simulink model "adaptive_control_sim"  (R2020a)
settings: Solver=FixedStepAuto  StartTime=0.0  StopTime=T  FixedStep=dtmax  MaxStep=dtmax  RelTol=1e-3
values from neighbouring files (symbols this model uses):
  b = b*b_error_scale    (= 131.4)    [Hinf_run.m]    (also in adaptive_control_run.m; passivity_fmod_run.m; passivity_velmod_run.m)
  bhat = 100    [adaptive_control_run.m]
  fe_dz = 15    [adaptive_control_run.m]
  input_type = 3    [Hinf_run.m]    (also in adaptive_control_run.m; passivity_fmod_run.m; passivity_velmod_run.m)
  k = k*k_error_scale    (= 11691)    [Hinf_run.m]    (also in adaptive_control_run.m; passivity_fmod_run.m; passivity_velmod_run.m)
  Kb = 40    [adaptive_control_run.m]
  khat = 11000    [adaptive_control_run.m]
  KK = 40    [adaptive_control_run.m]
  m = 500    [Hinf_run.m]    (also in adaptive_control_run.m; passivity_fmod_run.m; passivity_velmod_run.m)
  rampslope = 0.1    [Hinf_run.m]    (also in adaptive_control_run.m; passivity_fmod_run.m; passivity_velmod_run.m)
  sineamp = 0.1    [Hinf_run.m]    (also in adaptive_control_run.m; passivity_fmod_run.m; passivity_velmod_run.m)
  sinefreq = pi/2    (= 1.57079632679)    [Hinf_run.m]    (also in adaptive_control_run.m; passivity_fmod_run.m; passivity_velmod_run.m)
  stepval = 0.1    [Hinf_run.m]    (also in adaptive_control_run.m; passivity_fmod_run.m; passivity_velmod_run.m)
  taum = taum*taum_error_scale    (= 0.108)    [Hinf_run.m]    (also in adaptive_control_run.m; passivity_fmod_run.m; passivity_velmod_run.m)
  taumreal = 1*taum    (= 0.108)    [adaptive_control_run.m]
settings Model: Creator=davidcarabis  LastModifiedBy=davidcarabis
settings DataIOCC: ReturnWorkspaceOutputs=off

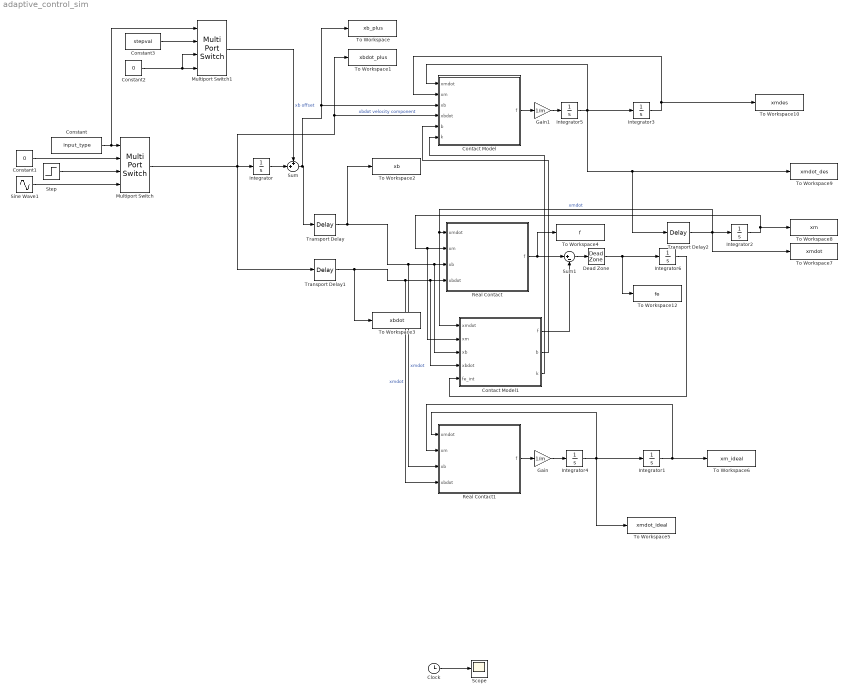
== system adaptive_control_sim ==
  Clock : Clock
  Constant : Constant  Value=input_type
  Constant1 : Constant  Value=0
  Constant2 : Constant  Value=0
  Constant3 : Constant  Value=stepval
  Contact Model : Subsystem
  Contact Model1 : Subsystem
  Dead Zone : DeadZone  LowerValue=-fe_dz  UpperValue=fe_dz  SaturateOnIntegerOverflow=on
  Gain : Gain  Gain=1/m
  Gain1 : Gain  Gain=1/m
  Integrator{,1..6} (7 alike) : Integrator
  Multiport Switch : MultiPortSwitch
  Multiport Switch1 : MultiPortSwitch
  Real Contact : Subsystem
  Real Contact1 : Subsystem
  Scope : Scope
  Sine Wave1 : Sin  Amplitude=sineamp*sinefreq  Frequency=sinefreq  Phase=pi/2  SampleTime=0
  Step : Step  Time=0  After=rampslope  SampleTime=0
  Sum : Sum  Inputs=++|
  Sum1 : Sum  Inputs=|+-
  To Workspace : ToWorkspace  VariableName=xb_plus
  To Workspace1 : ToWorkspace  VariableName=xbdot_plus
  To Workspace10 : ToWorkspace  VariableName=xmdes
  To Workspace12 : ToWorkspace  VariableName=fe
  To Workspace2 : ToWorkspace  VariableName=xb
  To Workspace3 : ToWorkspace  VariableName=xbdot
  To Workspace4 : ToWorkspace  VariableName=f
  To Workspace5 : ToWorkspace  VariableName=xmdot_ideal
  To Workspace6 : ToWorkspace  VariableName=xm_ideal
  To Workspace7 : ToWorkspace  VariableName=xmdot
  To Workspace8 : ToWorkspace  VariableName=xm
  To Workspace9 : ToWorkspace  VariableName=xmdot_des
  Transport Delay : TransportDelay  DelayTime=taum
  Transport Delay1 : TransportDelay  DelayTime=taum
  Transport Delay2 : TransportDelay  DelayTime=taumreal
  wires:
  Constant2/1 -> Multiport Switch1/3, Multiport Switch1/4
  Constant1/1 -> Multiport Switch/2
  Integrator/1 -> Sum/2
  Multiport Switch1/1 -> Sum/1  "xb offset"
  Constant/1 -> Multiport Switch1/1, Multiport Switch/1
  Multiport Switch/1 -> Transport Delay1/1, Contact Model/4(xbdot), To Workspace1/1, Integrator/1  "xbdot velocity component"
  Sine Wave1/1 -> Multiport Switch/4
  Step/1 -> Multiport Switch/3
  Constant3/1 -> Multiport Switch1/2
  Sum/1 -> Contact Model/3(xb), To Workspace/1, Transport Delay/1
  Transport Delay/1 -> To Workspace2/1, Contact Model1/3(xb), Real Contact/3(xb), Real Contact1/3(xb)  "xmdot"
  Transport Delay1/1 -> To Workspace3/1, Contact Model1/4(xbdot), Real Contact/4(xbdot), Real Contact1/4(xbdot)  "xmdot"
  Integrator5/1 -> Contact Model/1(xmdot), Integrator3/1, To Workspace9/1, Transport Delay2/1
  Integrator3/1 -> Contact Model/2(xm), To Workspace10/1
  Transport Delay2/1 -> Contact Model1/1(xmdot), Real Contact/1(xmdot), Integrator2/1, To Workspace7/1  "xmdot"
  Integrator2/1 -> Contact Model1/2(xm), Real Contact/2(xm), To Workspace8/1
  Real Contact1/1(f) -> Gain/1
  Integrator4/1 -> Integrator1/1, To Workspace5/1, Real Contact1/1(xmdot)
  Integrator1/1 -> To Workspace6/1, Real Contact1/2(xm)
  Gain/1 -> Integrator4/1
  Gain1/1 -> Integrator5/1
  Contact Model/1(f) -> Gain1/1
  Real Contact/1(f) -> Sum1/1, To Workspace4/1
  Sum1/1 -> Dead Zone/1
  Contact Model1/1(f) -> Sum1/2
  Contact Model1/2(b) -> Contact Model/5(b)
  Contact Model1/3(k) -> Contact Model/6(k)
  Integrator6/1 -> Contact Model1/5(fe_int)
  Clock/1 -> Scope/1
  Dead Zone/1 -> To Workspace12/1, Integrator6/1

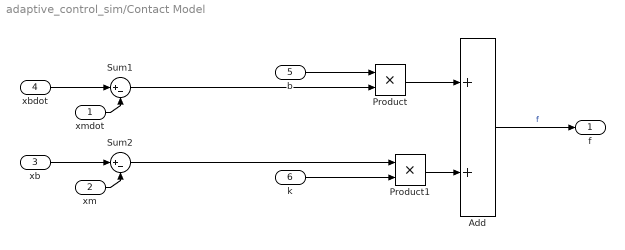
== system adaptive_control_sim/Contact Model ==
  xmdot : Inport
  xm : Inport  Port=2
  xb : Inport  Port=3
  xbdot : Inport  Port=4
  b : Inport  Port=5
  k : Inport  Port=6
  Add : Sum
  Product : Product
  Product1 : Product
  Sum1 : Sum  Inputs=|+-
  Sum2 : Sum  Inputs=|+-
  f : Outport  VectorParamsAs1DForOutWhenUnconnected=off
  wires:
  xmdot/1 -> Sum1/2
  Add/1 -> f/1  "f"
  xb/1 -> Sum2/1
  Product1/1 -> Add/2
  Sum1/1 -> Product/2
  xbdot/1 -> Sum1/1
  Product/1 -> Add/1
  xm/1 -> Sum2/2
  Sum2/1 -> Product1/1
  b/1 -> Product/1
  k/1 -> Product1/2

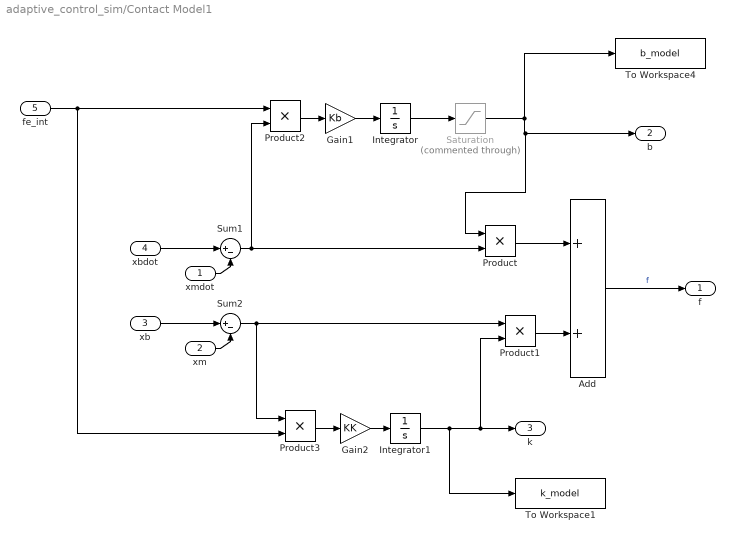
== system adaptive_control_sim/Contact Model1 ==
  xmdot : Inport
  xm : Inport  Port=2
  xb : Inport  Port=3
  xbdot : Inport  Port=4
  fe_int : Inport  Port=5
  Add : Sum
  Gain1 : Gain  Gain=Kb
  Gain2 : Gain  Gain=KK
  Integrator : Integrator  InitialCondition=bhat
  Integrator1 : Integrator  InitialCondition=khat
  Product{,1..3} (4 alike) : Product
  Saturation : Saturate  Commented=through  UpperLimit=Inf  LowerLimit=0
  Sum1 : Sum  Inputs=|+-
  Sum2 : Sum  Inputs=|+-
  To Workspace1 : ToWorkspace  VariableName=k_model
  To Workspace4 : ToWorkspace  VariableName=b_model
  f : Outport  VectorParamsAs1DForOutWhenUnconnected=off
  b : Outport  Port=2  VectorParamsAs1DForOutWhenUnconnected=off
  k : Outport  Port=3  VectorParamsAs1DForOutWhenUnconnected=off
  wires:
  xmdot/1 -> Sum1/2
  Add/1 -> f/1  "f"
  xb/1 -> Sum2/1
  Product1/1 -> Add/2
  Sum1/1 -> Product/2, Product2/2
  xbdot/1 -> Sum1/1
  Product/1 -> Add/1
  xm/1 -> Sum2/2
  Integrator/1 -> Saturation/1
  fe_int/1 -> Product3/2, Product2/1
  Sum2/1 -> Product1/1, Product3/1
  Integrator1/1 -> To Workspace1/1, k/1, Product1/2
  Product2/1 -> Gain1/1
  Gain1/1 -> Integrator/1
  Product3/1 -> Gain2/1
  Gain2/1 -> Integrator1/1
  Saturation/1 -> b/1, Product/1, To Workspace4/1

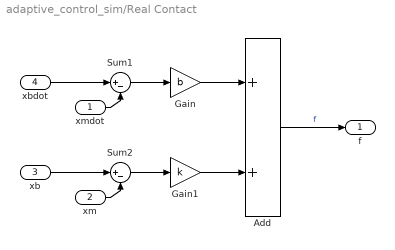
== system adaptive_control_sim/Real Contact ==
  xmdot : Inport
  xm : Inport  Port=2
  xb : Inport  Port=3
  xbdot : Inport  Port=4
  Add : Sum
  Gain : Gain  Gain=b
  Gain1 : Gain  Gain=k
  Sum1 : Sum  Inputs=|+-
  Sum2 : Sum  Inputs=|+-
  f : Outport  VectorParamsAs1DForOutWhenUnconnected=off
  wires:
  xmdot/1 -> Sum1/2
  Add/1 -> f/1  "f"
  Sum2/1 -> Gain1/1
  xb/1 -> Sum2/1
  Gain1/1 -> Add/2
  Sum1/1 -> Gain/1
  xbdot/1 -> Sum1/1
  Gain/1 -> Add/1
  xm/1 -> Sum2/2

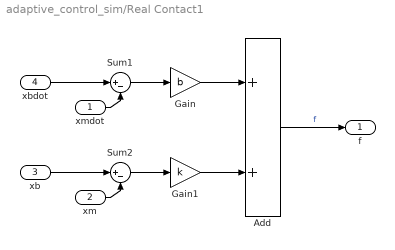
== system adaptive_control_sim/Real Contact1 ==
  xmdot : Inport
  xm : Inport  Port=2
  xb : Inport  Port=3
  xbdot : Inport  Port=4
  Add : Sum
  Gain : Gain  Gain=b
  Gain1 : Gain  Gain=k
  Sum1 : Sum  Inputs=|+-
  Sum2 : Sum  Inputs=|+-
  f : Outport  VectorParamsAs1DForOutWhenUnconnected=off
  wires:
  xmdot/1 -> Sum1/2
  Add/1 -> f/1  "f"
  Sum2/1 -> Gain1/1
  xb/1 -> Sum2/1
  Gain1/1 -> Add/2
  Sum1/1 -> Gain/1
  xbdot/1 -> Sum1/1
  Gain/1 -> Add/1
  xm/1 -> Sum2/2
